simulink model "sim_battery_system"  (R2018b)
settings: Solver=FixedStepDiscrete  StartTime=0.0  StopTime=SimPara.t_sim  FixedStep=SimPara.t_step  RelTol=1e-3
undefined symbols (not defined in the file or in its folder): A, BatPara, i, LSAPara, p, SimPara, SysPara, x2_cal, x3_cal, x_cal
libraries: simulink x14, dspstat3 x4, dspindex x1
(part 3 of 4)

== system sim_battery_system/Monitoring and Logging/Load Spectrum Analysis/Load Spectrum Analysis ON/Load Spectrum Analysis ON/One parametric LSA of cell delta temperature ==
  data_in : Inport
  For Iterator val1 : Subsystem  TreatAsAtomicUnit=on
  delay for selector data input : UnitDelay  SampleTime=-1
  LSA_out : Outport
  wires:
  data_in/1 -> For Iterator val1/1(data_in)
  For Iterator val1/1(LSA_out) -> delay for selector data input/1, LSA_out/1
  delay for selector data input/1 -> For Iterator val1/2(data_in_delay)

== system sim_battery_system/Monitoring and Logging/Load Spectrum Analysis/Load Spectrum Analysis ON/Load Spectrum Analysis ON/One parametric LSA of cell temperatures ==
  data_in : Inport
  For Iterator val1 : Subsystem  TreatAsAtomicUnit=on
  delay for selector data input : UnitDelay  SampleTime=-1
  LSA_out : Outport
  wires:
  data_in/1 -> For Iterator val1/1(data_in)
  For Iterator val1/1(LSA_out) -> delay for selector data input/1, LSA_out/1
  delay for selector data input/1 -> For Iterator val1/2(data_in_delay)

== system sim_battery_system/Monitoring and Logging/Load Spectrum Analysis/Load Spectrum Analysis ON/Load Spectrum Analysis ON/Subsystem1 ==
  In1 : Inport
  Clock : Clock
  Compare To Constant : simulink/Logic and Bit Operations/Compare To Constant  relop=>=  const=start/100 * SimPara.t_sim  OutDataTypeStr=boolean
  SubsyMMatrssdatrixm : Subsystem
  Out1 : Outport
  wires:
  Clock/1 -> Compare To Constant/1
  Compare To Constant/1 -> SubsyMMatrssdatrixm/Enable
  SubsyMMatrssdatrixm/1(Out1) -> Out1/1
  In1/1 -> SubsyMMatrssdatrixm/1(In1)

== system sim_battery_system/Monitoring and Logging/Load Spectrum Analysis/Load Spectrum Analysis ON/Load Spectrum Analysis ON/Subsystem2 ==
  In1 : Inport
  Clock : Clock
  Compare To Constant : simulink/Logic and Bit Operations/Compare To Constant  relop=>=  const=start/100 * SimPara.t_sim  OutDataTypeStr=boolean
  SubsyMMatrssdatrixm : Subsystem
  Out1 : Outport
  wires:
  In1/1 -> SubsyMMatrssdatrixm/1(In1)
  SubsyMMatrssdatrixm/1(Out1) -> Out1/1
  Compare To Constant/1 -> SubsyMMatrssdatrixm/Enable
  Clock/1 -> Compare To Constant/1

== system sim_battery_system/Monitoring and Logging/Load Spectrum Analysis/Load Spectrum Analysis ON/Load Spectrum Analysis ON/Subsystem3 ==
  In1 : Inport
  Clock : Clock
  Compare To Constant : simulink/Logic and Bit Operations/Compare To Constant  relop=>=  const=start/100 * SimPara.t_sim  OutDataTypeStr=boolean
  SubsyMMatrssdatrixm : Subsystem
  Out1 : Outport
  wires:
  Clock/1 -> Compare To Constant/1
  Compare To Constant/1 -> SubsyMMatrssdatrixm/Enable
  SubsyMMatrssdatrixm/1(Out1) -> Out1/1
  In1/1 -> SubsyMMatrssdatrixm/1(In1)

== system sim_battery_system/Monitoring and Logging/Load Spectrum Analysis/Load Spectrum Analysis ON/Load Spectrum Analysis ON/Subsystem4 ==
  In1 : Inport
  Clock : Clock
  Compare To Constant : simulink/Logic and Bit Operations/Compare To Constant  relop=>=  const=start/100 * SimPara.t_sim  OutDataTypeStr=boolean
  SubsyMMatrssdatrixm : Subsystem
  Out1 : Outport
  wires:
  In1/1 -> SubsyMMatrssdatrixm/1(In1)
  SubsyMMatrssdatrixm/1(Out1) -> Out1/1
  Compare To Constant/1 -> SubsyMMatrssdatrixm/Enable
  Clock/1 -> Compare To Constant/1

== system sim_battery_system/Monitoring and Logging/Load Spectrum Analysis/Load Spectrum Analysis ON/Load Spectrum Analysis ON/Subsystem5 ==
  In1 : Inport
  Clock : Clock
  Compare To Constant : simulink/Logic and Bit Operations/Compare To Constant  relop=>=  const=start/100 * SimPara.t_sim  OutDataTypeStr=boolean
  SubsyMMatrssdatrixm : Subsystem
  Out1 : Outport
  wires:
  Clock/1 -> Compare To Constant/1
  Compare To Constant/1 -> SubsyMMatrssdatrixm/Enable
  SubsyMMatrssdatrixm/1(Out1) -> Out1/1
  In1/1 -> SubsyMMatrssdatrixm/1(In1)

== system sim_battery_system/Monitoring and Logging/Load Spectrum Analysis/Load Spectrum Analysis ON/Load Spectrum Analysis ON/Subsystem6 ==
  In1 : Inport
  Clock : Clock
  Compare To Constant : simulink/Logic and Bit Operations/Compare To Constant  relop=>=  const=start/100 * SimPara.t_sim  OutDataTypeStr=boolean
  SubsyMMatrssdatrixm : Subsystem
  Out1 : Outport
  wires:
  In1/1 -> SubsyMMatrssdatrixm/1(In1)
  SubsyMMatrssdatrixm/1(Out1) -> Out1/1
  Compare To Constant/1 -> SubsyMMatrssdatrixm/Enable
  Clock/1 -> Compare To Constant/1

== system sim_battery_system/Monitoring and Logging/Load Spectrum Analysis/Load Spectrum Analysis ON/Load Spectrum Analysis ON/Subsystem7 ==
  In1 : Inport
  Clock : Clock
  Compare To Constant : simulink/Logic and Bit Operations/Compare To Constant  relop=>=  const=start/100 * SimPara.t_sim  OutDataTypeStr=boolean
  SubsyMMatrssdatrixm : Subsystem
  Out1 : Outport
  wires:
  Clock/1 -> Compare To Constant/1
  Compare To Constant/1 -> SubsyMMatrssdatrixm/Enable
  SubsyMMatrssdatrixm/1(Out1) -> Out1/1
  In1/1 -> SubsyMMatrssdatrixm/1(In1)

== system sim_battery_system/Monitoring and Logging/Load Spectrum Analysis/Load Spectrum Analysis ON/Load Spectrum Analysis ON/Subsystem8 ==
  In1 : Inport
  Clock : Clock
  Compare To Constant : simulink/Logic and Bit Operations/Compare To Constant  relop=>=  const=start/100 * SimPara.t_sim  OutDataTypeStr=boolean
  SubsyMMatrssdatrixm : Subsystem
  Out1 : Outport
  wires:
  Clock/1 -> Compare To Constant/1
  Compare To Constant/1 -> SubsyMMatrssdatrixm/Enable
  SubsyMMatrssdatrixm/1(Out1) -> Out1/1
  In1/1 -> SubsyMMatrssdatrixm/1(In1)

== system sim_battery_system/Monitoring and Logging/Load Spectrum Analysis/Load Spectrum Analysis ON/Load Spectrum Analysis ON/Subsystem9 ==
  In1 : Inport
  Clock : Clock
  Compare To Constant : simulink/Logic and Bit Operations/Compare To Constant  relop=>=  const=start/100 * SimPara.t_sim  OutDataTypeStr=boolean
  SubsyMMatrssdatrixm : Subsystem
  Out1 : Outport
  wires:
  In1/1 -> SubsyMMatrssdatrixm/1(In1)
  SubsyMMatrssdatrixm/1(Out1) -> Out1/1
  Compare To Constant/1 -> SubsyMMatrssdatrixm/Enable
  Clock/1 -> Compare To Constant/1

== system sim_battery_system/Monitoring and Logging/Load Spectrum Analysis/Load Spectrum Analysis ON/Load Spectrum Analysis ON/Two parametric LSA of cell C-Rate vs. temperature ==
  val1_in : Inport
  val2_in : Inport  Port=2
  For Iterator val1 : Subsystem  TreatAsAtomicUnit=on
  delay for selector data input : UnitDelay  SampleTime=-1
  LSA_out : Outport
  wires:
  val2_in/1 -> For Iterator val1/2(val_2_in)
  val1_in/1 -> For Iterator val1/1(val1_in)
  For Iterator val1/1(LSA_out) -> LSA_out/1, delay for selector data input/1
  delay for selector data input/1 -> For Iterator val1/3(data_in_delayed)

== system sim_battery_system/Monitoring and Logging/Load Spectrum Analysis/Load Spectrum Analysis ON/Load Spectrum Analysis ON/Two parametric LSA of cell SOC vs. C-Rate ==
  val1_in : Inport
  val2_in : Inport  Port=2
  For Iterator val1 : Subsystem  TreatAsAtomicUnit=on
  delay for selector data input : UnitDelay  SampleTime=-1
  LSA_out : Outport
  wires:
  delay for selector data input/1 -> For Iterator val1/3(data_in_delayed)
  For Iterator val1/1(LSA_out) -> delay for selector data input/1, LSA_out/1
  val1_in/1 -> For Iterator val1/1(val1_in)
  val2_in/1 -> For Iterator val1/2(val_2_in)

== system sim_battery_system/Monitoring and Logging/Load Spectrum Analysis/Load Spectrum Analysis ON/Load Spectrum Analysis ON/Two parametric LSA of cell SOC vs. temperature  ==
  val1_in : Inport
  val2_in : Inport  Port=2
  For Iterator val1 : Subsystem  TreatAsAtomicUnit=on
  delay for selector data input : UnitDelay  SampleTime=-1
  LSA_out : Outport
  wires:
  delay for selector data input/1 -> For Iterator val1/3(data_in_delayed)
  For Iterator val1/1(LSA_out) -> delay for selector data input/1, LSA_out/1
  val1_in/1 -> For Iterator val1/1(val1_in)
  val2_in/1 -> For Iterator val1/2(val_2_in)

== system sim_battery_system/Monitoring and Logging/Temperature Sensor Simulation/Enable//disable temperature sensors/TempSensors ON/Iterate through the sensors ==
  note: Save sensor value in vector
  note: Get T_cell values for sensor
  note: Exclude zeros
  note: Select row of sensor
  note: Matrix with cell IDs for each sensor
  T_cells_vec : Inport
  Assignment : Assignment  DiagnosticForDimensions=Warning  IndexOptions=Index vector (port)  Indices=Sensor1  OutputSizes=1
  Constant : Constant  Value=SysPara.thermal.sensors.sensor_mat  VectorParams1D=off
  Find Nonzero Elements : Find  NumberOfInputDimensions=3  IndexMode=Zero-based  ShowOutputForNonzeroInputValues=on
  For Iterator : ForIterator  IterationLimit=size(SysPara.thermal.sensors.sensor_mat,1)
  Mean : dspstat3/Mean  run=off  InputProcessing=Columns as channels (frame based)  reset_popup=None  directionMode=Entire input  dimension=1  roiEnable=off  roiType=Rectangles  roiPortion=Entire ROI  roiOutput=Individual statistics for each ROI  roiFlag=off  roundingMode=Floor  overflowMode=off  outputDataTypeStr=Inherit: Same as accumulator  outputMin=[]  outputMax=[]  outputLastDataTypeStr=Inherit: Same as accumulator
  Memory : Memory  InitialCondition=zeros(size(SysPara.thermal.sensors.sensor_mat,1),1)  InheritSampleTime=on
  Selector1 : Selector  NumberOfDimensions=2  InputPortWidth=sn  IndexOptions=Index vector (port),Select all  Indices=A(i),1  OutputSizes=1,1
  Selector2 : Selector  InputPortWidth=SysPara.p * SysPara.s  IndexOptions=Index vector (port)  Indices=[1 3]  OutputSizes=1
  Terminator : Terminator
  T_sensors [°C] : Outport
  wires:
  For Iterator/1 -> Selector1/2, Assignment/3
  T_cells_vec/1 -> Selector2/1
  Selector2/1 -> Mean/1
  Assignment/1 -> T_sensors [°C]/1, Memory/1
  Mean/1 -> Assignment/2
  Memory/1 -> Assignment/1
  Constant/1 -> Selector1/1
  Selector1/1 -> Find Nonzero Elements/1
  Find Nonzero Elements/2 -> Selector2/2
  Find Nonzero Elements/1 -> Terminator/1

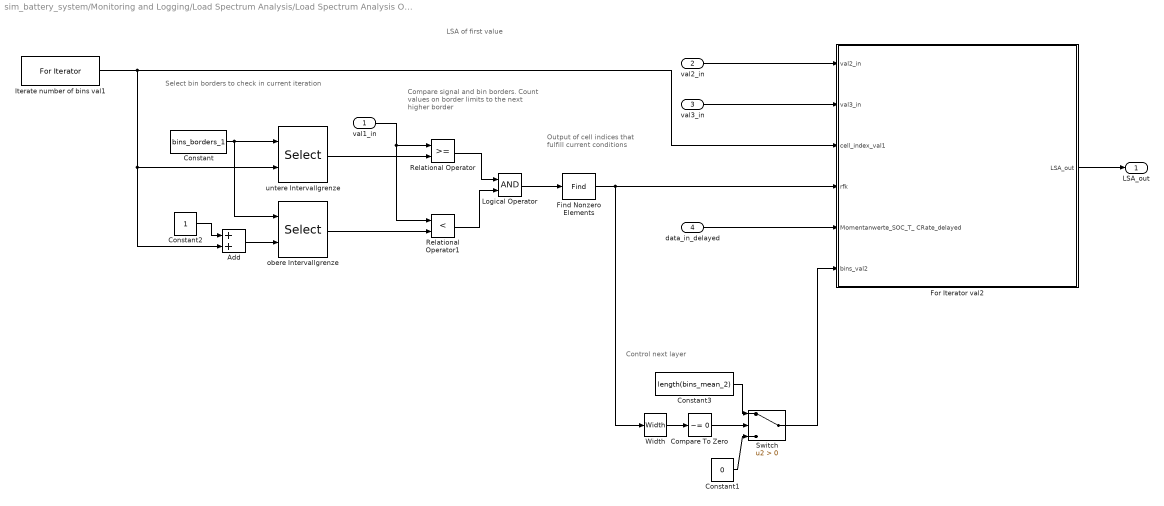
== system sim_battery_system/Monitoring and Logging/Load Spectrum Analysis/Load Spectrum Analysis ON/Load Spectrum Analysis ON/3-parametrische Momentanwertzählung SOC, T_Cells, CRate/For Iterator val1 ==
  note: Select bin borders to check in current iteration
  note: Output of cell indices that fulfill current conditions
  note: Compare signal and bin borders. Count values on border limits to the next higher border
  note: LSA of first value
  note: Control next layer
  val1_in : Inport
  val2_in : Inport  Port=2
  val3_in : Inport  Port=3
  data_in_delayed : Inport  Port=4
  Add : Sum
  Compare To Zero : simulink/Logic and Bit Operations/Compare To Zero  relop=~=  OutDataTypeStr=boolean
  Constant : Constant  Value=bins_borders_1
  Constant1 : Constant  Value=0
  Constant2 : Constant
  Constant3 : Constant  Value=length(bins_mean_2)
  Find Nonzero Elements : Find
  For Iterator val2 : Subsystem  TreatAsAtomicUnit=on
  Iterate number of bins val1 : ForIterator  ResetStates=reset  IterationLimit=length(bins_mean_1)  IterationVariableDataType=double
  Logical Operator : Logic  AllPortsSameDT=off  OutDataTypeStr=boolean
  Relational Operator : RelationalOperator  OutDataTypeStr=boolean  RndMeth=Simplest
  Relational Operator1 : RelationalOperator  Operator=<  OutDataTypeStr=boolean  RndMeth=Simplest
  Switch : Switch  Criteria=u2 > Threshold
  Width : Width
  obere Intervallgrenze : Selector  InputPortWidth=length(bins_borders_1)  IndexOptions=Index vector (port)  Indices=1:p  OutputSizes=1
  untere Intervallgrenze : Selector  InputPortWidth=length(bins_borders_1)  IndexOptions=Index vector (port)  Indices=1:p  OutputSizes=1
  LSA_out : Outport
  wires:
  Switch/1 -> For Iterator val2/6(bins_val2)
  Constant3/1 -> Switch/1
  Width/1 -> Compare To Zero/1
  Constant1/1 -> Switch/3
  Compare To Zero/1 -> Switch/2
  Find Nonzero Elements/1 -> For Iterator val2/4(rfk), Width/1
  val3_in/1 -> For Iterator val2/2(val3_in)
  val2_in/1 -> For Iterator val2/1(val2_in)
  Logical Operator/1 -> Find Nonzero Elements/1
  Relational Operator/1 -> Logical Operator/1
  Relational Operator1/1 -> Logical Operator/2
  val1_in/1 -> Relational Operator/1, Relational Operator1/1
  obere Intervallgrenze/1 -> Relational Operator1/2
  untere Intervallgrenze/1 -> Relational Operator/2
  Iterate number of bins val1/1 -> For Iterator val2/3(cell_index_val1), untere Intervallgrenze/2, Add/2
  Constant2/1 -> Add/1
  Add/1 -> obere Intervallgrenze/2
  Constant/1 -> untere Intervallgrenze/1, obere Intervallgrenze/1
  For Iterator val2/1(LSA_out) -> LSA_out/1
  data_in_delayed/1 -> For Iterator val2/5(Momentanwerte_SOC_T_ CRate_delayed)

== system sim_battery_system/Monitoring and Logging/Load Spectrum Analysis/Load Spectrum Analysis ON/Load Spectrum Analysis ON/One parametric LSA of cell C-Rate/For Iterator val1 ==
  data_in : Inport
  data_in_delay : Inport  Port=2
  Add : Sum
  Assignment Subsystem : Subsystem  TreatAsAtomicUnit=on
  Constant : Constant  Value=bins_borders
  Constant2 : Constant
  Find Nonzero Elements : Find
  Iterate number of bins : ForIterator  ResetStates=reset  IterationLimit=length(bins_mean)  IterationVariableDataType=double
  Logical Operator : Logic  AllPortsSameDT=off  OutDataTypeStr=boolean
  Relational Operator : RelationalOperator  OutDataTypeStr=boolean  RndMeth=Simplest
  Relational Operator1 : RelationalOperator  Operator=<  OutDataTypeStr=boolean  RndMeth=Simplest
  select bin upper border : Selector  InputPortWidth=length(bins_borders)  IndexOptions=Index vector (port)  Indices=1:p  OutputSizes=1
  select parallel cell2 : Selector  InputPortWidth=length(bins_borders)  IndexOptions=Index vector (port)  Indices=1:p  OutputSizes=1
  LSA_out : Outport
  wires:
  Assignment Subsystem/1(LSA_out) -> LSA_out/1
  Find Nonzero Elements/1 -> Assignment Subsystem/2(index_cell)
  Logical Operator/1 -> Find Nonzero Elements/1
  Relational Operator/1 -> Logical Operator/1
  Relational Operator1/1 -> Logical Operator/2
  data_in/1 -> Relational Operator/1, Relational Operator1/1
  select bin upper border/1 -> Relational Operator1/2
  select parallel cell2/1 -> Relational Operator/2
  Iterate number of bins/1 -> select parallel cell2/2, Assignment Subsystem/1(k), Add/2
  Constant2/1 -> Add/1
  Add/1 -> select bin upper border/2
  Constant/1 -> select parallel cell2/1, select bin upper border/1
  data_in_delay/1 -> Assignment Subsystem/3(data_in_delayed)

== system sim_battery_system/Monitoring and Logging/Load Spectrum Analysis/Load Spectrum Analysis ON/Load Spectrum Analysis ON/One parametric LSA of cell SOC/For Iterator val1 ==
  data_in : Inport
  data_in_delay : Inport  Port=2
  Add : Sum
  Assignment Subsystem : Subsystem  TreatAsAtomicUnit=on
  Constant : Constant  Value=bins_borders
  Constant2 : Constant
  Find Nonzero Elements : Find
  Iterate number of bins : ForIterator  ResetStates=reset  IterationLimit=length(bins_mean)  IterationVariableDataType=double
  Logical Operator : Logic  AllPortsSameDT=off  OutDataTypeStr=boolean
  Relational Operator : RelationalOperator  OutDataTypeStr=boolean  RndMeth=Simplest
  Relational Operator1 : RelationalOperator  Operator=<  OutDataTypeStr=boolean  RndMeth=Simplest
  select bin upper border : Selector  InputPortWidth=length(bins_borders)  IndexOptions=Index vector (port)  Indices=1:p  OutputSizes=1
  select parallel cell2 : Selector  InputPortWidth=length(bins_borders)  IndexOptions=Index vector (port)  Indices=1:p  OutputSizes=1
  LSA_out : Outport
  wires:
  data_in_delay/1 -> Assignment Subsystem/3(data_in_delayed)
  Constant/1 -> select bin upper border/1, select parallel cell2/1
  Add/1 -> select bin upper border/2
  Constant2/1 -> Add/1
  Iterate number of bins/1 -> Add/2, Assignment Subsystem/1(k), select parallel cell2/2
  select parallel cell2/1 -> Relational Operator/2
  select bin upper border/1 -> Relational Operator1/2
  data_in/1 -> Relational Operator1/1, Relational Operator/1
  Relational Operator1/1 -> Logical Operator/2
  Relational Operator/1 -> Logical Operator/1
  Logical Operator/1 -> Find Nonzero Elements/1
  Find Nonzero Elements/1 -> Assignment Subsystem/2(index_cell)
  Assignment Subsystem/1(LSA_out) -> LSA_out/1

== system sim_battery_system/Monitoring and Logging/Load Spectrum Analysis/Load Spectrum Analysis ON/Load Spectrum Analysis ON/One parametric LSA of cell delta C-Rate/For Iterator val1 ==
  data_in : Inport
  data_in_delay : Inport  Port=2
  Add : Sum
  Assignment Subsystem : Subsystem  TreatAsAtomicUnit=on
  Constant : Constant  Value=bins_borders
  Constant2 : Constant
  Find Nonzero Elements : Find
  Iterate number of bins : ForIterator  ResetStates=reset  IterationLimit=length(bins_mean)  IterationVariableDataType=double
  Logical Operator : Logic  AllPortsSameDT=off  OutDataTypeStr=boolean
  Relational Operator : RelationalOperator  OutDataTypeStr=boolean  RndMeth=Simplest
  Relational Operator1 : RelationalOperator  Operator=<  OutDataTypeStr=boolean  RndMeth=Simplest
  select bin upper border : Selector  InputPortWidth=length(bins_borders)  IndexOptions=Index vector (port)  Indices=1:p  OutputSizes=1
  select parallel cell2 : Selector  InputPortWidth=length(bins_borders)  IndexOptions=Index vector (port)  Indices=1:p  OutputSizes=1
  LSA_out : Outport
  wires:
  data_in_delay/1 -> Assignment Subsystem/3(data_in_delayed)
  Constant/1 -> select bin upper border/1, select parallel cell2/1
  Add/1 -> select bin upper border/2
  Constant2/1 -> Add/1
  Iterate number of bins/1 -> Add/2, Assignment Subsystem/1(k), select parallel cell2/2
  select parallel cell2/1 -> Relational Operator/2
  select bin upper border/1 -> Relational Operator1/2
  data_in/1 -> Relational Operator1/1, Relational Operator/1
  Relational Operator1/1 -> Logical Operator/2
  Relational Operator/1 -> Logical Operator/1
  Logical Operator/1 -> Find Nonzero Elements/1
  Find Nonzero Elements/1 -> Assignment Subsystem/2(index_cell)
  Assignment Subsystem/1(LSA_out) -> LSA_out/1

== system sim_battery_system/Monitoring and Logging/Load Spectrum Analysis/Load Spectrum Analysis ON/Load Spectrum Analysis ON/One parametric LSA of cell delta temperature/For Iterator val1 ==
  data_in : Inport
  data_in_delay : Inport  Port=2
  Add : Sum
  Assignment Subsystem : Subsystem  TreatAsAtomicUnit=on
  Constant : Constant  Value=bins_borders
  Constant2 : Constant
  Find Nonzero Elements : Find
  Iterate number of bins : ForIterator  ResetStates=reset  IterationLimit=length(bins_mean)  IterationVariableDataType=double
  Logical Operator : Logic  AllPortsSameDT=off  OutDataTypeStr=boolean
  Relational Operator : RelationalOperator  OutDataTypeStr=boolean  RndMeth=Simplest
  Relational Operator1 : RelationalOperator  Operator=<  OutDataTypeStr=boolean  RndMeth=Simplest
  select bin upper border : Selector  InputPortWidth=length(bins_borders)  IndexOptions=Index vector (port)  Indices=1:p  OutputSizes=1
  select parallel cell2 : Selector  InputPortWidth=length(bins_borders)  IndexOptions=Index vector (port)  Indices=1:p  OutputSizes=1
  LSA_out : Outport
  wires:
  Assignment Subsystem/1(LSA_out) -> LSA_out/1
  Find Nonzero Elements/1 -> Assignment Subsystem/2(index_cell)
  Logical Operator/1 -> Find Nonzero Elements/1
  Relational Operator/1 -> Logical Operator/1
  Relational Operator1/1 -> Logical Operator/2
  data_in/1 -> Relational Operator/1, Relational Operator1/1
  select bin upper border/1 -> Relational Operator1/2
  select parallel cell2/1 -> Relational Operator/2
  Iterate number of bins/1 -> select parallel cell2/2, Assignment Subsystem/1(k), Add/2
  Constant2/1 -> Add/1
  Add/1 -> select bin upper border/2
  Constant/1 -> select parallel cell2/1, select bin upper border/1
  data_in_delay/1 -> Assignment Subsystem/3(data_in_delayed)

== system sim_battery_system/Monitoring and Logging/Load Spectrum Analysis/Load Spectrum Analysis ON/Load Spectrum Analysis ON/One parametric LSA of cell temperatures/For Iterator val1 ==
  data_in : Inport
  data_in_delay : Inport  Port=2
  Add : Sum
  Assignment Subsystem : Subsystem  TreatAsAtomicUnit=on
  Constant : Constant  Value=bins_borders
  Constant2 : Constant
  Find Nonzero Elements : Find
  Iterate number of bins : ForIterator  ResetStates=reset  IterationLimit=length(bins_mean)  IterationVariableDataType=double
  Logical Operator : Logic  AllPortsSameDT=off  OutDataTypeStr=boolean
  Relational Operator : RelationalOperator  OutDataTypeStr=boolean  RndMeth=Simplest
  Relational Operator1 : RelationalOperator  Operator=<  OutDataTypeStr=boolean  RndMeth=Simplest
  select bin upper border : Selector  InputPortWidth=length(bins_borders)  IndexOptions=Index vector (port)  Indices=1:p  OutputSizes=1
  select parallel cell2 : Selector  InputPortWidth=length(bins_borders)  IndexOptions=Index vector (port)  Indices=1:p  OutputSizes=1
  LSA_out : Outport
  wires:
  Assignment Subsystem/1(LSA_out) -> LSA_out/1
  Find Nonzero Elements/1 -> Assignment Subsystem/2(index_cell)
  Logical Operator/1 -> Find Nonzero Elements/1
  Relational Operator/1 -> Logical Operator/1
  Relational Operator1/1 -> Logical Operator/2
  data_in/1 -> Relational Operator/1, Relational Operator1/1
  select bin upper border/1 -> Relational Operator1/2
  select parallel cell2/1 -> Relational Operator/2
  Iterate number of bins/1 -> select parallel cell2/2, Assignment Subsystem/1(k), Add/2
  Constant2/1 -> Add/1
  Add/1 -> select bin upper border/2
  Constant/1 -> select parallel cell2/1, select bin upper border/1
  data_in_delay/1 -> Assignment Subsystem/3(data_in_delayed)

== system sim_battery_system/Monitoring and Logging/Load Spectrum Analysis/Load Spectrum Analysis ON/Load Spectrum Analysis ON/Subsystem1/SubsyMMatrssdatrixm ==
  In1 : Inport
  Enable : EnablePort  PropagateVarSize=During execution
  "summiert Dim. 4, die die Einzelzelle angibt" : Sum  Inputs=+  CollapseMode=Specified dimension  CollapseDim=dim
  Out1 : Outport
  wires:
  In1/1 -> "summiert Dim. 4, die die Einzelzelle angibt"/1
  "summiert Dim. 4, die die Einzelzelle angibt"/1 -> Out1/1

== system sim_battery_system/Monitoring and Logging/Load Spectrum Analysis/Load Spectrum Analysis ON/Load Spectrum Analysis ON/Subsystem2/SubsyMMatrssdatrixm ==
  In1 : Inport
  Enable : EnablePort  PropagateVarSize=During execution
  "summiert Dim. 4, die die Einzelzelle angibt" : Sum  Inputs=+  CollapseMode=Specified dimension  CollapseDim=dim
  Out1 : Outport
  wires:
  "summiert Dim. 4, die die Einzelzelle angibt"/1 -> Out1/1
  In1/1 -> "summiert Dim. 4, die die Einzelzelle angibt"/1

== system sim_battery_system/Monitoring and Logging/Load Spectrum Analysis/Load Spectrum Analysis ON/Load Spectrum Analysis ON/Subsystem3/SubsyMMatrssdatrixm ==
  In1 : Inport
  Enable : EnablePort  PropagateVarSize=During execution
  "summiert Dim. 4, die die Einzelzelle angibt" : Sum  Inputs=+  CollapseMode=Specified dimension  CollapseDim=dim
  Out1 : Outport
  wires:
  In1/1 -> "summiert Dim. 4, die die Einzelzelle angibt"/1
  "summiert Dim. 4, die die Einzelzelle angibt"/1 -> Out1/1

== system sim_battery_system/Monitoring and Logging/Load Spectrum Analysis/Load Spectrum Analysis ON/Load Spectrum Analysis ON/Subsystem4/SubsyMMatrssdatrixm ==
  In1 : Inport
  Enable : EnablePort  PropagateVarSize=During execution
  "summiert Dim. 4, die die Einzelzelle angibt" : Sum  Inputs=+  CollapseMode=Specified dimension  CollapseDim=dim
  Out1 : Outport
  wires:
  "summiert Dim. 4, die die Einzelzelle angibt"/1 -> Out1/1
  In1/1 -> "summiert Dim. 4, die die Einzelzelle angibt"/1

== system sim_battery_system/Monitoring and Logging/Load Spectrum Analysis/Load Spectrum Analysis ON/Load Spectrum Analysis ON/Subsystem5/SubsyMMatrssdatrixm ==
  In1 : Inport
  Enable : EnablePort  PropagateVarSize=During execution
  "summiert Dim. 4, die die Einzelzelle angibt" : Sum  Inputs=+  CollapseMode=Specified dimension  CollapseDim=dim
  Out1 : Outport
  wires:
  In1/1 -> "summiert Dim. 4, die die Einzelzelle angibt"/1
  "summiert Dim. 4, die die Einzelzelle angibt"/1 -> Out1/1

== system sim_battery_system/Monitoring and Logging/Load Spectrum Analysis/Load Spectrum Analysis ON/Load Spectrum Analysis ON/Subsystem6/SubsyMMatrssdatrixm ==
  In1 : Inport
  Enable : EnablePort  PropagateVarSize=During execution
  "summiert Dim. 4, die die Einzelzelle angibt" : Sum  Inputs=+  CollapseMode=Specified dimension  CollapseDim=dim
  Out1 : Outport
  wires:
  "summiert Dim. 4, die die Einzelzelle angibt"/1 -> Out1/1
  In1/1 -> "summiert Dim. 4, die die Einzelzelle angibt"/1

== system sim_battery_system/Monitoring and Logging/Load Spectrum Analysis/Load Spectrum Analysis ON/Load Spectrum Analysis ON/Subsystem7/SubsyMMatrssdatrixm ==
  In1 : Inport
  Enable : EnablePort  PropagateVarSize=During execution
  "summiert Dim. 4, die die Einzelzelle angibt" : Sum  Inputs=+  CollapseMode=Specified dimension  CollapseDim=dim
  Out1 : Outport
  wires:
  In1/1 -> "summiert Dim. 4, die die Einzelzelle angibt"/1
  "summiert Dim. 4, die die Einzelzelle angibt"/1 -> Out1/1

== system sim_battery_system/Monitoring and Logging/Load Spectrum Analysis/Load Spectrum Analysis ON/Load Spectrum Analysis ON/Subsystem8/SubsyMMatrssdatrixm ==
  In1 : Inport
  Enable : EnablePort  PropagateVarSize=During execution
  "summiert Dim. 4, die die Einzelzelle angibt" : Sum  Inputs=+  CollapseMode=Specified dimension  CollapseDim=dim
  Out1 : Outport
  wires:
  In1/1 -> "summiert Dim. 4, die die Einzelzelle angibt"/1
  "summiert Dim. 4, die die Einzelzelle angibt"/1 -> Out1/1

== system sim_battery_system/Monitoring and Logging/Load Spectrum Analysis/Load Spectrum Analysis ON/Load Spectrum Analysis ON/Subsystem9/SubsyMMatrssdatrixm ==
  In1 : Inport
  Enable : EnablePort  PropagateVarSize=During execution
  "summiert Dim. 4, die die Einzelzelle angibt" : Sum  Inputs=+  CollapseMode=Specified dimension  CollapseDim=dim
  Out1 : Outport
  wires:
  "summiert Dim. 4, die die Einzelzelle angibt"/1 -> Out1/1
  In1/1 -> "summiert Dim. 4, die die Einzelzelle angibt"/1

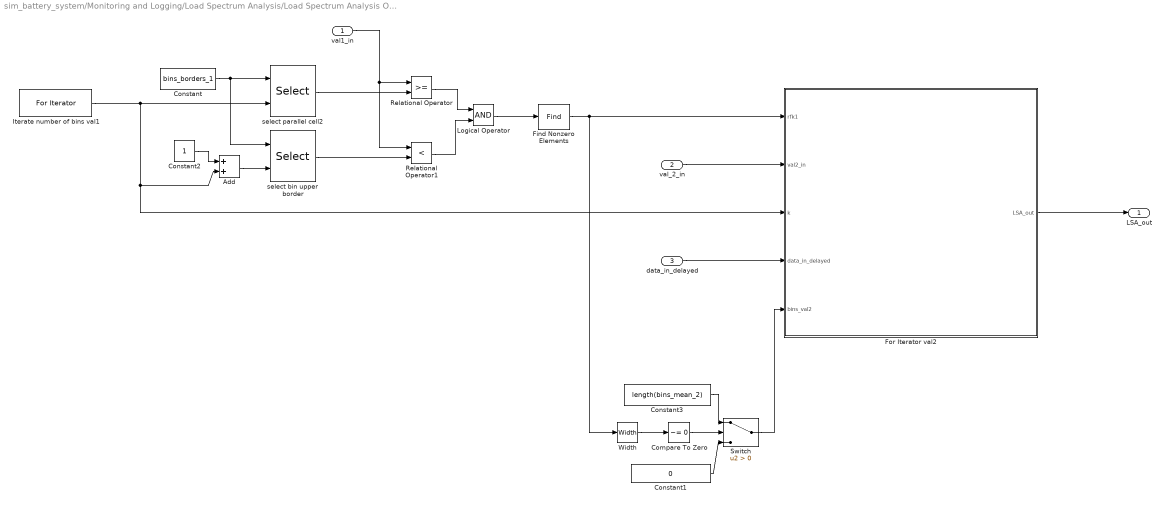
== system sim_battery_system/Monitoring and Logging/Load Spectrum Analysis/Load Spectrum Analysis ON/Load Spectrum Analysis ON/Two parametric LSA of cell C-Rate vs. temperature/For Iterator val1 ==
  val1_in : Inport
  val_2_in : Inport  Port=2
  data_in_delayed : Inport  Port=3
  Add : Sum
  Compare To Zero : simulink/Logic and Bit Operations/Compare To Zero  relop=~=  OutDataTypeStr=boolean
  Constant : Constant  Value=bins_borders_1
  Constant1 : Constant  Value=0
  Constant2 : Constant
  Constant3 : Constant  Value=length(bins_mean_2)
  Find Nonzero Elements : Find
  "For Iterator val2 " : Subsystem  TreatAsAtomicUnit=on
  Iterate number of bins val1 : ForIterator  ResetStates=reset  IterationLimit=length(bins_mean_1)  IterationVariableDataType=double
  Logical Operator : Logic  AllPortsSameDT=off  OutDataTypeStr=boolean
  Relational Operator : RelationalOperator  OutDataTypeStr=boolean  RndMeth=Simplest
  Relational Operator1 : RelationalOperator  Operator=<  OutDataTypeStr=boolean  RndMeth=Simplest
  Switch : Switch  Criteria=u2 > Threshold
  Width : Width
  select bin upper border : Selector  InputPortWidth=length(bins_borders_1)  IndexOptions=Index vector (port)  Indices=1:p  OutputSizes=1
  select parallel cell2 : Selector  InputPortWidth=length(bins_borders_1)  IndexOptions=Index vector (port)  Indices=1:p  OutputSizes=1
  LSA_out : Outport
  wires:
  val_2_in/1 -> "For Iterator val2 "/2(val2_in)
  Find Nonzero Elements/1 -> "For Iterator val2 "/1(rfk1), Width/1
  Logical Operator/1 -> Find Nonzero Elements/1
  Relational Operator/1 -> Logical Operator/1
  Relational Operator1/1 -> Logical Operator/2
  val1_in/1 -> Relational Operator/1, Relational Operator1/1
  select bin upper border/1 -> Relational Operator1/2
  select parallel cell2/1 -> Relational Operator/2
  Iterate number of bins val1/1 -> select parallel cell2/2, Add/2, "For Iterator val2 "/3(k)
  Constant2/1 -> Add/1
  Add/1 -> select bin upper border/2
  Constant/1 -> select parallel cell2/1, select bin upper border/1
  "For Iterator val2 "/1(LSA_out) -> LSA_out/1
  data_in_delayed/1 -> "For Iterator val2 "/4(data_in_delayed)
  Compare To Zero/1 -> Switch/2
  Constant1/1 -> Switch/3
  Width/1 -> Compare To Zero/1
  Switch/1 -> "For Iterator val2 "/5(bins_val2)
  Constant3/1 -> Switch/1

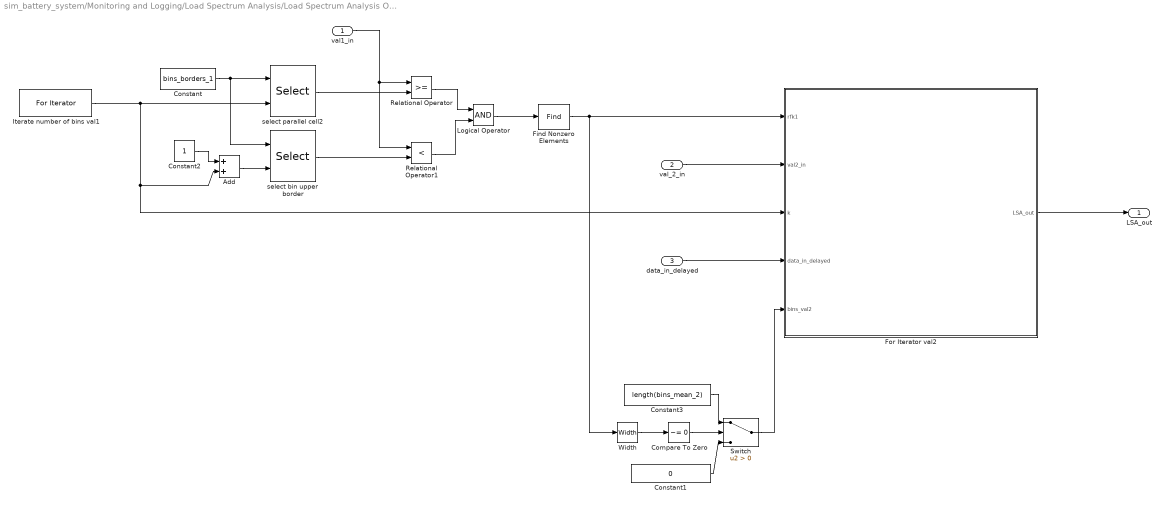
== system sim_battery_system/Monitoring and Logging/Load Spectrum Analysis/Load Spectrum Analysis ON/Load Spectrum Analysis ON/Two parametric LSA of cell SOC vs. C-Rate/For Iterator val1 ==
  val1_in : Inport
  val_2_in : Inport  Port=2
  data_in_delayed : Inport  Port=3
  Add : Sum
  Compare To Zero : simulink/Logic and Bit Operations/Compare To Zero  relop=~=  OutDataTypeStr=boolean
  Constant : Constant  Value=bins_borders_1
  Constant1 : Constant  Value=0
  Constant2 : Constant
  Constant3 : Constant  Value=length(bins_mean_2)
  Find Nonzero Elements : Find
  "For Iterator val2 " : Subsystem  TreatAsAtomicUnit=on
  Iterate number of bins val1 : ForIterator  ResetStates=reset  IterationLimit=length(bins_mean_1)  IterationVariableDataType=double
  Logical Operator : Logic  AllPortsSameDT=off  OutDataTypeStr=boolean
  Relational Operator : RelationalOperator  OutDataTypeStr=boolean  RndMeth=Simplest
  Relational Operator1 : RelationalOperator  Operator=<  OutDataTypeStr=boolean  RndMeth=Simplest
  Switch : Switch  Criteria=u2 > Threshold
  Width : Width
  select bin upper border : Selector  InputPortWidth=length(bins_borders_1)  IndexOptions=Index vector (port)  Indices=1:p  OutputSizes=1
  select parallel cell2 : Selector  InputPortWidth=length(bins_borders_1)  IndexOptions=Index vector (port)  Indices=1:p  OutputSizes=1
  LSA_out : Outport
  wires:
  Constant3/1 -> Switch/1
  Switch/1 -> "For Iterator val2 "/5(bins_val2)
  Width/1 -> Compare To Zero/1
  Constant1/1 -> Switch/3
  Compare To Zero/1 -> Switch/2
  data_in_delayed/1 -> "For Iterator val2 "/4(data_in_delayed)
  "For Iterator val2 "/1(LSA_out) -> LSA_out/1
  Constant/1 -> select bin upper border/1, select parallel cell2/1
  Add/1 -> select bin upper border/2
  Constant2/1 -> Add/1
  Iterate number of bins val1/1 -> "For Iterator val2 "/3(k), Add/2, select parallel cell2/2
  select parallel cell2/1 -> Relational Operator/2
  select bin upper border/1 -> Relational Operator1/2
  val1_in/1 -> Relational Operator1/1, Relational Operator/1
  Relational Operator1/1 -> Logical Operator/2
  Relational Operator/1 -> Logical Operator/1
  Logical Operator/1 -> Find Nonzero Elements/1
  Find Nonzero Elements/1 -> Width/1, "For Iterator val2 "/1(rfk1)
  val_2_in/1 -> "For Iterator val2 "/2(val2_in)

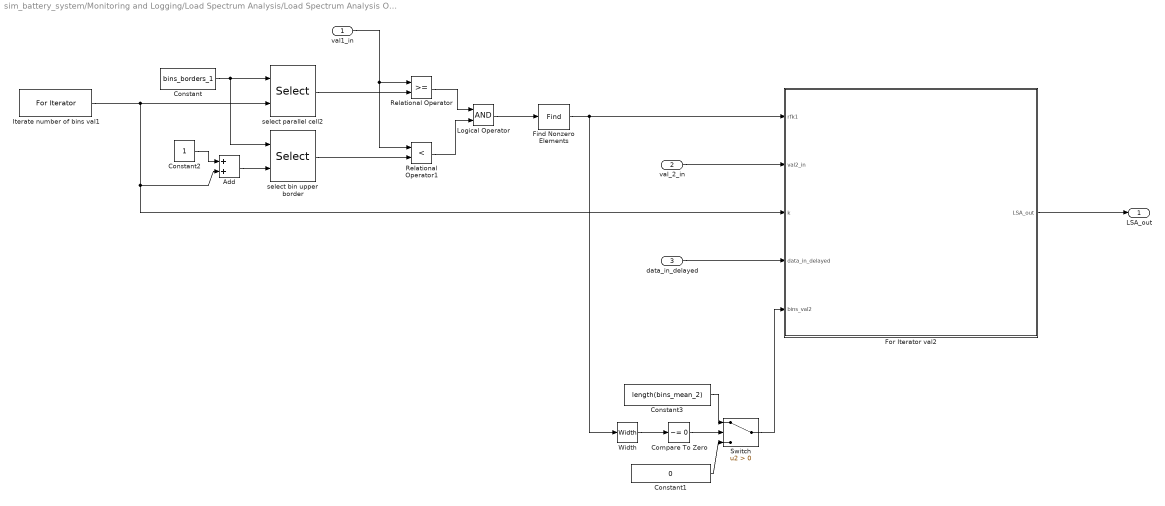
== system sim_battery_system/Monitoring and Logging/Load Spectrum Analysis/Load Spectrum Analysis ON/Load Spectrum Analysis ON/Two parametric LSA of cell SOC vs. temperature /For Iterator val1 ==
  val1_in : Inport
  val_2_in : Inport  Port=2
  data_in_delayed : Inport  Port=3
  Add : Sum
  Compare To Zero : simulink/Logic and Bit Operations/Compare To Zero  relop=~=  OutDataTypeStr=boolean
  Constant : Constant  Value=bins_borders_1
  Constant1 : Constant  Value=0
  Constant2 : Constant
  Constant3 : Constant  Value=length(bins_mean_2)
  Find Nonzero Elements : Find
  "For Iterator val2 " : Subsystem  TreatAsAtomicUnit=on
  Iterate number of bins val1 : ForIterator  ResetStates=reset  IterationLimit=length(bins_mean_1)  IterationVariableDataType=double
  Logical Operator : Logic  AllPortsSameDT=off  OutDataTypeStr=boolean
  Relational Operator : RelationalOperator  OutDataTypeStr=boolean  RndMeth=Simplest
  Relational Operator1 : RelationalOperator  Operator=<  OutDataTypeStr=boolean  RndMeth=Simplest
  Switch : Switch  Criteria=u2 > Threshold
  Width : Width
  select bin upper border : Selector  InputPortWidth=length(bins_borders_1)  IndexOptions=Index vector (port)  Indices=1:p  OutputSizes=1
  select parallel cell2 : Selector  InputPortWidth=length(bins_borders_1)  IndexOptions=Index vector (port)  Indices=1:p  OutputSizes=1
  LSA_out : Outport
  wires:
  Constant3/1 -> Switch/1
  Switch/1 -> "For Iterator val2 "/5(bins_val2)
  Width/1 -> Compare To Zero/1
  Constant1/1 -> Switch/3
  Compare To Zero/1 -> Switch/2
  data_in_delayed/1 -> "For Iterator val2 "/4(data_in_delayed)
  "For Iterator val2 "/1(LSA_out) -> LSA_out/1
  Constant/1 -> select bin upper border/1, select parallel cell2/1
  Add/1 -> select bin upper border/2
  Constant2/1 -> Add/1
  Iterate number of bins val1/1 -> "For Iterator val2 "/3(k), Add/2, select parallel cell2/2
  select parallel cell2/1 -> Relational Operator/2
  select bin upper border/1 -> Relational Operator1/2
  val1_in/1 -> Relational Operator1/1, Relational Operator/1
  Relational Operator1/1 -> Logical Operator/2
  Relational Operator/1 -> Logical Operator/1
  Logical Operator/1 -> Find Nonzero Elements/1
  Find Nonzero Elements/1 -> Width/1, "For Iterator val2 "/1(rfk1)
  val_2_in/1 -> "For Iterator val2 "/2(val2_in)

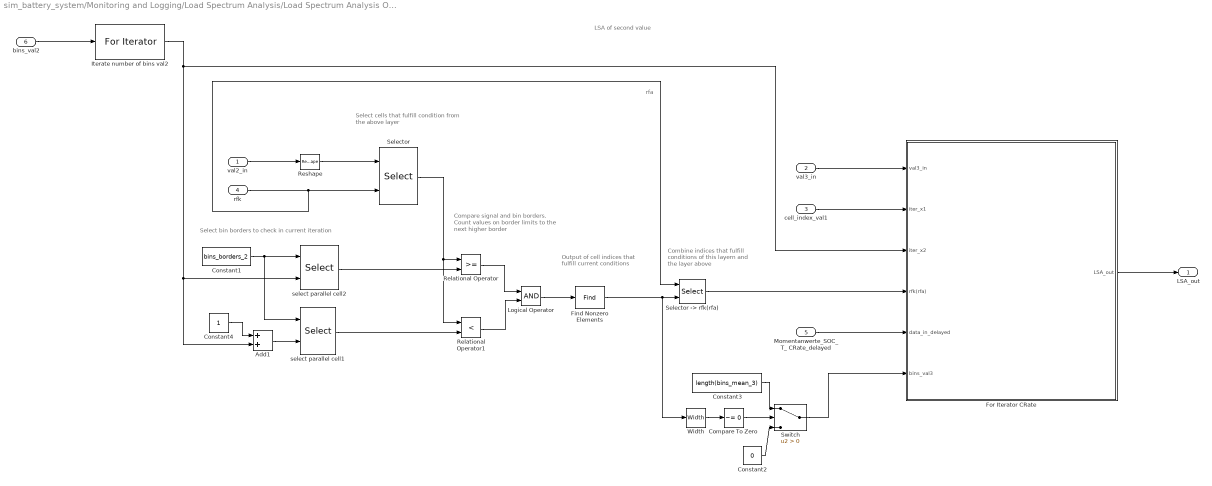
== system sim_battery_system/Monitoring and Logging/Load Spectrum Analysis/Load Spectrum Analysis ON/Load Spectrum Analysis ON/3-parametrische Momentanwertzählung SOC, T_Cells, CRate/For Iterator val1/For Iterator val2 ==
  note: Select cells that fulfill condition from the above layer
  note: LSA of second value
  note: rfa
  note: Select bin borders to check in current iteration
  note: Compare signal and bin borders. Count values on border limits to the next higher border
  note: Output of cell indices that fulfill current conditions
  note: Combine indices that fulfill conditions of this layern and the layer above
  val2_in : Inport
  val3_in : Inport  Port=2
  cell_index_val1 : Inport  Port=3
  rfk : Inport  Port=4
  Momentanwerte_SOC_T_ CRate_delayed : Inport  Port=5
  bins_val2 : Inport  Port=6
  Add1 : Sum
  Compare To Zero : simulink/Logic and Bit Operations/Compare To Zero  relop=~=  OutDataTypeStr=boolean
  Constant1 : Constant  Value=bins_borders_2
  Constant2 : Constant  Value=0
  Constant3 : Constant  Value=length(bins_mean_3)
  Constant4 : Constant
  Find Nonzero Elements : Find
  For Iterator CRate : Subsystem  TreatAsAtomicUnit=on
  Iterate number of bins val2 : ForIterator  ResetStates=reset  IterationSource=external  IterationLimit=length(x2_cal)  IterationVariableDataType=double
  Logical Operator : Logic  AllPortsSameDT=off  OutDataTypeStr=boolean
  Relational Operator : RelationalOperator  OutDataTypeStr=boolean  RndMeth=Simplest
  Relational Operator1 : RelationalOperator  Operator=<  OutDataTypeStr=boolean  RndMeth=Simplest
  Reshape : Reshape
  Selector : Selector  InputPortWidth=SysPara.p*SysPara.s  IndexOptions=Index vector (port)  Indices=1:p  OutputSizes=1
  "Selector -> rfk(rfa)" : Selector  InputPortWidth=SysPara.p*SysPara.s  IndexOptions=Index vector (port)  Indices=[1 3]  OutputSizes=1
  Switch : Switch  Criteria=u2 > Threshold
  Width : Width
  select parallel cell1 : Selector  InputPortWidth=length(bins_borders_2)  IndexOptions=Index vector (port)  Indices=1:p  OutputSizes=1
  select parallel cell2 : Selector  InputPortWidth=length(bins_borders_2)  IndexOptions=Index vector (port)  Indices=1:p  OutputSizes=1
  LSA_out : Outport
  wires:
  Switch/1 -> For Iterator CRate/6(bins_val3)
  Constant3/1 -> Switch/1
  Width/1 -> Compare To Zero/1
  Constant2/1 -> Switch/3
  Compare To Zero/1 -> Switch/2
  Find Nonzero Elements/1 -> "Selector -> rfk(rfa)"/2, Width/1
  bins_val2/1 -> Iterate number of bins val2/1
  val3_in/1 -> For Iterator CRate/1(val3_in)
  For Iterator CRate/1(LSA_out) -> LSA_out/1
  "Selector -> rfk(rfa)"/1 -> For Iterator CRate/4(rfk(rfa))
  rfk/1 -> Selector/2, "Selector -> rfk(rfa)"/1
  Logical Operator/1 -> Find Nonzero Elements/1
  Reshape/1 -> Selector/1
  val2_in/1 -> Reshape/1
  cell_index_val1/1 -> For Iterator CRate/2(iter_x1)
  Selector/1 -> Relational Operator/1, Relational Operator1/1
  Relational Operator/1 -> Logical Operator/1
  Relational Operator1/1 -> Logical Operator/2
  select parallel cell1/1 -> Relational Operator1/2
  select parallel cell2/1 -> Relational Operator/2
  Constant4/1 -> Add1/1
  Add1/1 -> select parallel cell1/2
  Iterate number of bins val2/1 -> select parallel cell2/2, Add1/2, For Iterator CRate/3(iter_x2)
  Constant1/1 -> select parallel cell2/1, select parallel cell1/1
  Momentanwerte_SOC_T_ CRate_delayed/1 -> For Iterator CRate/5(data_in_delayed)

== system sim_battery_system/Monitoring and Logging/Load Spectrum Analysis/Load Spectrum Analysis ON/Load Spectrum Analysis ON/One parametric LSA of cell C-Rate/For Iterator val1/Assignment Subsystem ==
  k : Inport
  index_cell : Inport  Port=2
  data_in_delayed : Inport  Port=3
  Add : Sum
  Assignment of matrix entries : Assignment  NumberOfDimensions=2  OutputInitialize=Specify size for each dimension in table  IndexOptions=Index vector (port),Index vector (port)  Indices=1,1  OutputSizes=length(bins_mean),SysPara.p*SysPara.s+1
  Constant1 : Constant  Value=SimPara.t_step
  "Selection of delayed matrix entries " : Selector  NumberOfDimensions=2  InputPortWidth=3  IndexOptions=Index vector (port),Index vector (port)  Indices=[1 3],1  OutputSizes=1,1
  LSA_out : Outport
  wires:
  index_cell/1 -> Assignment of matrix entries/3, "Selection of delayed matrix entries "/3
  Assignment of matrix entries/1 -> LSA_out/1
  k/1 -> "Selection of delayed matrix entries "/2, Assignment of matrix entries/2
  Constant1/1 -> Add/1
  "Selection of delayed matrix entries "/1 -> Add/2
  Add/1 -> Assignment of matrix entries/1
  data_in_delayed/1 -> "Selection of delayed matrix entries "/1

== system sim_battery_system/Monitoring and Logging/Load Spectrum Analysis/Load Spectrum Analysis ON/Load Spectrum Analysis ON/One parametric LSA of cell SOC/For Iterator val1/Assignment Subsystem ==
  k : Inport
  index_cell : Inport  Port=2
  data_in_delayed : Inport  Port=3
  Add : Sum
  Assignment of matrix entries : Assignment  NumberOfDimensions=2  OutputInitialize=Specify size for each dimension in table  IndexOptions=Index vector (port),Index vector (port)  Indices=1,1  OutputSizes=length(bins_mean),SysPara.p*SysPara.s+1
  Constant1 : Constant  Value=SimPara.t_step
  "Selection of delayed matrix entries " : Selector  NumberOfDimensions=2  InputPortWidth=3  IndexOptions=Index vector (port),Index vector (port)  Indices=[1 3],1  OutputSizes=1,1
  LSA_out : Outport
  wires:
  data_in_delayed/1 -> "Selection of delayed matrix entries "/1
  Add/1 -> Assignment of matrix entries/1
  "Selection of delayed matrix entries "/1 -> Add/2
  Constant1/1 -> Add/1
  k/1 -> Assignment of matrix entries/2, "Selection of delayed matrix entries "/2
  Assignment of matrix entries/1 -> LSA_out/1
  index_cell/1 -> "Selection of delayed matrix entries "/3, Assignment of matrix entries/3

== system sim_battery_system/Monitoring and Logging/Load Spectrum Analysis/Load Spectrum Analysis ON/Load Spectrum Analysis ON/One parametric LSA of cell delta C-Rate/For Iterator val1/Assignment Subsystem ==
  k : Inport
  index_cell : Inport  Port=2
  data_in_delayed : Inport  Port=3
  Add : Sum
  Assignment of matrix entries : Assignment  NumberOfDimensions=2  OutputInitialize=Specify size for each dimension in table  IndexOptions=Index vector (port),Index vector (port)  Indices=1,1  OutputSizes=length(bins_mean),SysPara.p*SysPara.s+1
  Constant1 : Constant  Value=SimPara.t_step
  "Selection of delayed matrix entries " : Selector  NumberOfDimensions=2  InputPortWidth=3  IndexOptions=Index vector (port),Index vector (port)  Indices=[1 3],1  OutputSizes=1,1
  LSA_out : Outport
  wires:
  data_in_delayed/1 -> "Selection of delayed matrix entries "/1
  Add/1 -> Assignment of matrix entries/1
  "Selection of delayed matrix entries "/1 -> Add/2
  Constant1/1 -> Add/1
  k/1 -> Assignment of matrix entries/2, "Selection of delayed matrix entries "/2
  Assignment of matrix entries/1 -> LSA_out/1
  index_cell/1 -> "Selection of delayed matrix entries "/3, Assignment of matrix entries/3

== system sim_battery_system/Monitoring and Logging/Load Spectrum Analysis/Load Spectrum Analysis ON/Load Spectrum Analysis ON/One parametric LSA of cell delta temperature/For Iterator val1/Assignment Subsystem ==
  k : Inport
  index_cell : Inport  Port=2
  data_in_delayed : Inport  Port=3
  Add : Sum
  Assignment of matrix entries : Assignment  NumberOfDimensions=2  OutputInitialize=Specify size for each dimension in table  IndexOptions=Index vector (port),Index vector (port)  Indices=1,1  OutputSizes=length(bins_mean),SysPara.p*SysPara.s+1
  Constant1 : Constant  Value=SimPara.t_step
  "Selection of delayed matrix entries " : Selector  NumberOfDimensions=2  InputPortWidth=3  IndexOptions=Index vector (port),Index vector (port)  Indices=[1 3],1  OutputSizes=1,1
  LSA_out : Outport
  wires:
  index_cell/1 -> Assignment of matrix entries/3, "Selection of delayed matrix entries "/3
  Assignment of matrix entries/1 -> LSA_out/1
  k/1 -> "Selection of delayed matrix entries "/2, Assignment of matrix entries/2
  Constant1/1 -> Add/1
  "Selection of delayed matrix entries "/1 -> Add/2
  Add/1 -> Assignment of matrix entries/1
  data_in_delayed/1 -> "Selection of delayed matrix entries "/1

== system sim_battery_system/Monitoring and Logging/Load Spectrum Analysis/Load Spectrum Analysis ON/Load Spectrum Analysis ON/One parametric LSA of cell temperatures/For Iterator val1/Assignment Subsystem ==
  k : Inport
  index_cell : Inport  Port=2
  data_in_delayed : Inport  Port=3
  Add : Sum
  Assignment of matrix entries : Assignment  NumberOfDimensions=2  OutputInitialize=Specify size for each dimension in table  IndexOptions=Index vector (port),Index vector (port)  Indices=1,1  OutputSizes=length(bins_mean),SysPara.p*SysPara.s+1
  Constant1 : Constant  Value=SimPara.t_step
  "Selection of delayed matrix entries " : Selector  NumberOfDimensions=2  InputPortWidth=3  IndexOptions=Index vector (port),Index vector (port)  Indices=[1 3],1  OutputSizes=1,1
  LSA_out : Outport
  wires:
  index_cell/1 -> Assignment of matrix entries/3, "Selection of delayed matrix entries "/3
  Assignment of matrix entries/1 -> LSA_out/1
  k/1 -> "Selection of delayed matrix entries "/2, Assignment of matrix entries/2
  Constant1/1 -> Add/1
  "Selection of delayed matrix entries "/1 -> Add/2
  Add/1 -> Assignment of matrix entries/1
  data_in_delayed/1 -> "Selection of delayed matrix entries "/1

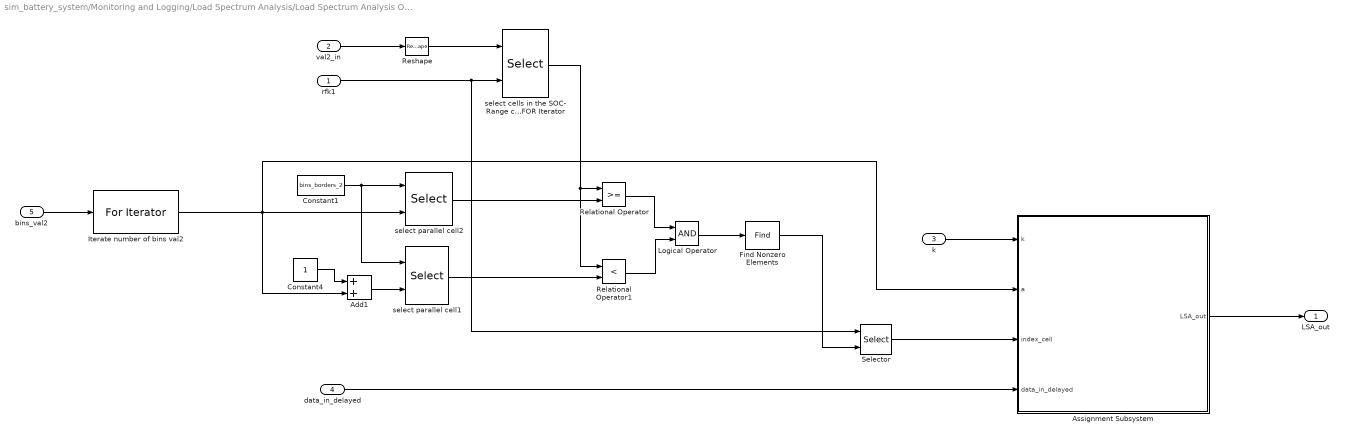
== system sim_battery_system/Monitoring and Logging/Load Spectrum Analysis/Load Spectrum Analysis ON/Load Spectrum Analysis ON/Two parametric LSA of cell C-Rate vs. temperature/For Iterator val1/For Iterator val2  ==
  rfk1 : Inport
  val2_in : Inport  Port=2
  k : Inport  Port=3
  data_in_delayed : Inport  Port=4
  bins_val2 : Inport  Port=5
  Add1 : Sum
  Assignment Subsystem : Subsystem  TreatAsAtomicUnit=on
  Constant1 : Constant  Value=bins_borders_2
  Constant4 : Constant
  Find Nonzero Elements : Find
  Iterate number of bins val2 : ForIterator  ResetStates=reset  IterationSource=external  IterationLimit=length(x_cal)  IterationVariableDataType=double
  Logical Operator : Logic  AllPortsSameDT=off  OutDataTypeStr=boolean
  Relational Operator : RelationalOperator  OutDataTypeStr=boolean  RndMeth=Simplest
  Relational Operator1 : RelationalOperator  Operator=<  OutDataTypeStr=boolean  RndMeth=Simplest
  Reshape : Reshape
  Selector : Selector  InputPortWidth=SysPara.p*SysPara.s  IndexOptions=Index vector (port)  Indices=[1 3]  OutputSizes=1
  select cells in the SOC- Range corresponding to 1. FOR Iterator : Selector  InputPortWidth=SysPara.p*SysPara.s  IndexOptions=Index vector (port)  Indices=1:p  OutputSizes=1
  select parallel cell1 : Selector  InputPortWidth=length(bins_borders_2)  IndexOptions=Index vector (port)  Indices=1:p  OutputSizes=1
  select parallel cell2 : Selector  InputPortWidth=length(bins_borders_2)  IndexOptions=Index vector (port)  Indices=1:p  OutputSizes=1
  LSA_out : Outport
  wires:
  Assignment Subsystem/1(LSA_out) -> LSA_out/1
  Selector/1 -> Assignment Subsystem/3(index_cell)
  Find Nonzero Elements/1 -> Selector/2
  rfk1/1 -> select cells in the SOC- Range corresponding to 1. FOR Iterator/2, Selector/1
  Logical Operator/1 -> Find Nonzero Elements/1
  Reshape/1 -> select cells in the SOC- Range corresponding to 1. FOR Iterator/1
  val2_in/1 -> Reshape/1
  k/1 -> Assignment Subsystem/1(k)
  select cells in the SOC- Range corresponding to 1. FOR Iterator/1 -> Relational Operator/1, Relational Operator1/1
  Relational Operator/1 -> Logical Operator/1
  Relational Operator1/1 -> Logical Operator/2
  select parallel cell1/1 -> Relational Operator1/2
  select parallel cell2/1 -> Relational Operator/2
  Constant4/1 -> Add1/1
  Add1/1 -> select parallel cell1/2
  Iterate number of bins val2/1 -> Add1/2, Assignment Subsystem/2(a), select parallel cell2/2
  Constant1/1 -> select parallel cell2/1, select parallel cell1/1
  data_in_delayed/1 -> Assignment Subsystem/4(data_in_delayed)
  bins_val2/1 -> Iterate number of bins val2/1

== system sim_battery_system/Monitoring and Logging/Load Spectrum Analysis/Load Spectrum Analysis ON/Load Spectrum Analysis ON/Two parametric LSA of cell SOC vs. C-Rate/For Iterator val1/For Iterator val2  ==
  rfk1 : Inport
  val2_in : Inport  Port=2
  k : Inport  Port=3
  data_in_delayed : Inport  Port=4
  bins_val2 : Inport  Port=5
  Add1 : Sum
  Assignment Subsystem : Subsystem  TreatAsAtomicUnit=on
  Constant1 : Constant  Value=bins_borders_2
  Constant4 : Constant
  Find Nonzero Elements : Find
  Iterate number of bins val2 : ForIterator  ResetStates=reset  IterationSource=external  IterationLimit=length(x_cal)  IterationVariableDataType=double
  Logical Operator : Logic  AllPortsSameDT=off  OutDataTypeStr=boolean
  Relational Operator : RelationalOperator  OutDataTypeStr=boolean  RndMeth=Simplest
  Relational Operator1 : RelationalOperator  Operator=<  OutDataTypeStr=boolean  RndMeth=Simplest
  Reshape : Reshape
  Selector : Selector  InputPortWidth=SysPara.p*SysPara.s  IndexOptions=Index vector (port)  Indices=[1 3]  OutputSizes=1
  select cells in the SOC- Range corresponding to 1. FOR Iterator : Selector  InputPortWidth=SysPara.p*SysPara.s  IndexOptions=Index vector (port)  Indices=1:p  OutputSizes=1
  select parallel cell1 : Selector  InputPortWidth=length(bins_borders_2)  IndexOptions=Index vector (port)  Indices=1:p  OutputSizes=1
  select parallel cell2 : Selector  InputPortWidth=length(bins_borders_2)  IndexOptions=Index vector (port)  Indices=1:p  OutputSizes=1
  LSA_out : Outport
  wires:
  bins_val2/1 -> Iterate number of bins val2/1
  data_in_delayed/1 -> Assignment Subsystem/4(data_in_delayed)
  Constant1/1 -> select parallel cell1/1, select parallel cell2/1
  Iterate number of bins val2/1 -> select parallel cell2/2, Assignment Subsystem/2(a), Add1/2
  Add1/1 -> select parallel cell1/2
  Constant4/1 -> Add1/1
  select parallel cell2/1 -> Relational Operator/2
  select parallel cell1/1 -> Relational Operator1/2
  Relational Operator1/1 -> Logical Operator/2
  Relational Operator/1 -> Logical Operator/1
  select cells in the SOC- Range corresponding to 1. FOR Iterator/1 -> Relational Operator1/1, Relational Operator/1
  k/1 -> Assignment Subsystem/1(k)
  val2_in/1 -> Reshape/1
  Reshape/1 -> select cells in the SOC- Range corresponding to 1. FOR Iterator/1
  Logical Operator/1 -> Find Nonzero Elements/1
  rfk1/1 -> Selector/1, select cells in the SOC- Range corresponding to 1. FOR Iterator/2
  Find Nonzero Elements/1 -> Selector/2
  Selector/1 -> Assignment Subsystem/3(index_cell)
  Assignment Subsystem/1(LSA_out) -> LSA_out/1
